simulink model "linecoordinate"  (R2022b)
settings: Solver=VariableStepAuto  StartTime=0.0  StopTime=1  RelTol=1e-3
settings Model: Creator=XinyiWu  LastModifiedBy=quanv

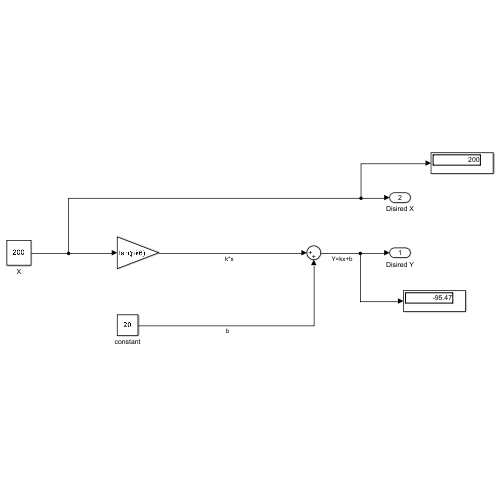
[thumbnail: Simulink's stored preview of the top-level diagram]
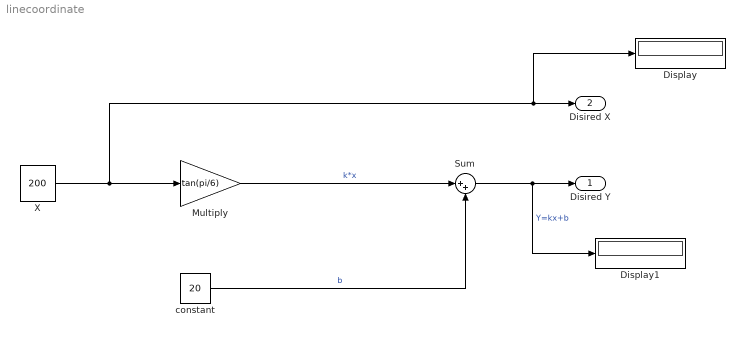
== system linecoordinate ==
  Display : Display
  Display1 : Display
  Multiply : Gain  Gain=tan(pi/6)
  Sum : Sum  Inputs=|++
  X : Constant  Value=200
  constant : Constant  Value=20
  Disired Y : Outport
  Disired X : Outport  Port=2
  wires:
  constant/1 -> Sum/2  "b"
  Sum/1 -> Display1/1, Disired Y/1  "Y=kx+b"
  Multiply/1 -> Sum/1  "k*x"
  X/1 -> Display/1, Disired X/1, Multiply/1
